simulink model "lab_2_1"  (R2023b)
settings: Solver=FixedStepAuto  StartTime=0.0  StopTime=10.0  FixedStep=0.001  RelTol=1e-3
undefined symbols (not defined in the file): a_0, a_1, dot_y_0, y_0
settings Model: Creator=nsukh  LastModifiedBy=nsukh

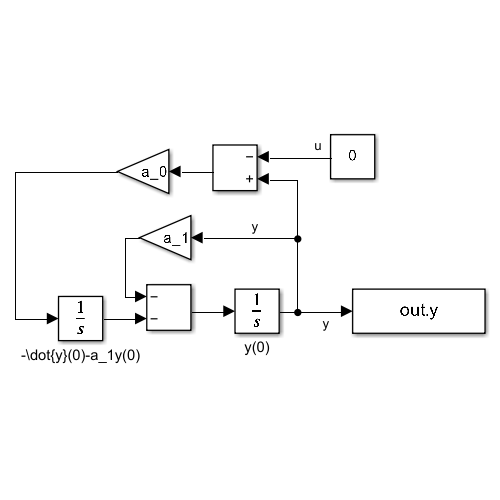
[thumbnail: Simulink's stored preview of the top-level diagram]
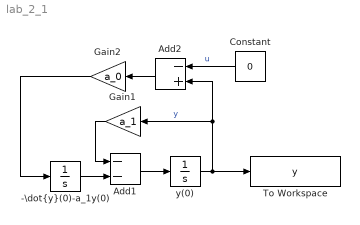
== system lab_2_1 ==
  "-\\dot{y}(0)-a_1y(0)" : Integrator  InitialCondition=-dot_y_0-a_1*y_0
  Add1 : Sum  Inputs=--
  Add2 : Sum  Inputs=-+
  Constant : Constant  Value=0  SampleTime=-1
  Gain1 : Gain  Gain=a_1
  Gain2 : Gain  Gain=a_0
  To Workspace : ToWorkspace  VariableName=y  SaveFormat=Timeseries  SampleTime=-1
  y(0) : Integrator  InitialCondition=y_0
  wires:
  Add1/1 -> y(0)/1
  Gain1/1 -> Add1/1
  "-\\dot{y}(0)-a_1y(0)"/1 -> Add1/2
  y(0)/1 -> To Workspace/1, Add2/2, Gain1/1  "y"
  Gain2/1 -> "-\\dot{y}(0)-a_1y(0)"/1
  Add2/1 -> Gain2/1
  Constant/1 -> Add2/1  "u"
